simulink model "RL_model"  (Simulink 7.4)
settings: Solver=ode45  StartTime=0.0  StopTime=0.05  RelTol=1e-7
settings Model: Creator=klu  LastModifiedBy=klu

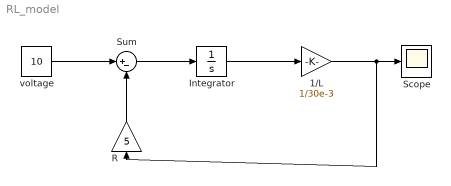
== system RL_model ==
  1/L : Gain  Gain=1/30e-3  ParameterDataType=fixdt(1, 16)  ParameterScaling=2^0  OutDataType=fixdt(1, 16)  OutScaling=2^0
  Integrator : Integrator
  R : Gain  Gain=5  ParameterDataType=fixdt(1, 16)  ParameterScaling=2^0  OutDataType=fixdt(1, 16)  OutScaling=2^0
  Scope : Scope
  Sum : Sum  Inputs=|+-  OutDataType=fixdt(1, 16)  OutScaling=2^0
  voltage : Constant  Value=10  OutDataType=fixdt(1, 16)  OutScaling=2^0
  wires:
  voltage/1 -> Sum/1
  R/1 -> Sum/2
  Sum/1 -> Integrator/1
  Integrator/1 -> 1/L/1
  1/L/1 -> Scope/1, R/1
